simulink model "Emergency_system"  (R2020a)
settings: Solver=ode23tb  StartTime=0.0  StopTime=20  RelTol=1e-4
undefined symbols (not defined in the file or in its folder): ee_sli_rtmsupport, gcbh
libraries: powerlib x10, sps_avr x7, simulink x3, powerlib_meascontrol x2, dspswit3 x1
settings Model: FPTRunName=Active  ExtModeTrigMode=oneshot  ExtModeArmWhenConnect=off  ExtModeAutoUpdateStatusClock=off  Creator=MathWorks  LastModifiedBy=assem
settings SolverCC: ZeroCrossAlgorithm=Adaptive
settings DataIOCC: SaveFormat=Array  SignalLoggingSaveFormat=ModelDataLogs  ReturnWorkspaceOutputs=off  SignalLoggingName=sigsOut  OutputTimes=[0:1/20:10]
settings OptimizationCC: BlockReduction=off  BooleanDataType=off  ExpressionDepthLimit=2147483647  InitFltsAndDblsToZero=on  EfficientMapNaN2IntZero=off  LifeSpan=inf
settings DebuggingCC: UnderspecifiedInitializationDetection=Classic  MergeDetectMultiDrivingBlocksExec=none  CheckExecutionContextPreStartOutputMsg=on  CheckExecutionContextRuntimeOutputMsg=on  SignalResolutionControl=TryResolveAllWithWarning  IgnoredZcDiagnostic=none  MultiTaskDSMMsg=warning  MultiTaskCondExecSysMsg=none  SigSpecEnsureSampleTimeMsg=none  FcnCallInpInsideContextMsg=warning  UnconnectedInputMsg=none  UnconnectedOutputMsg=none  UnconnectedLineMsg=none  StateNameClashWarn=warning  SFUnexpectedBacktrackingDiag=warning  SFNoUnconditionalDefaultTransitionDiag=warning  SFExecutionAtInitializationDiag=none  ArithmeticOperatorsInVariantConditions=warning
settings HardwareCC: ProdBitPerPointer=32  ProdBitPerSizeT=32  ProdBitPerPtrDiffT=32  ProdLargestAtomicFloat=None  ProdIntDivRoundTo=Undefined  ProdEndianess=Unspecified  ProdWordSize=32  ProdHWDeviceType=Specified  TargetUnknown=on
settings ModelReferenceCC: PropagateSignalLabelsOutOfModel=off
settings SFSimCC: SimUseLocalCustomCode=off  CustomCodeUndefinedFunction=UseInterfaceOnly
settings RTWCC: RTWUseLocalCustomCode=off
settings CodeAppCC: StateflowObjectComments=on
settings GRTTargetCC: TargetFcnLib=ansi_tfl_tmw.mat  TargetLangStandard=C89/C90 (ANSI)  CombineOutputUpdateFcns=off  GRTInterface=on
settings ConfigComp: CovMetricSettings=dw  CovHtmlReporting=on  CovSaveCumulativeToWorkspaceVar=on  CovSaveSingleToWorkspaceVar=on  CovExternalEMLEnable=off  CovSFcnEnable=off
settings SimscapeCC: SimscapeNormalizeSystem=off

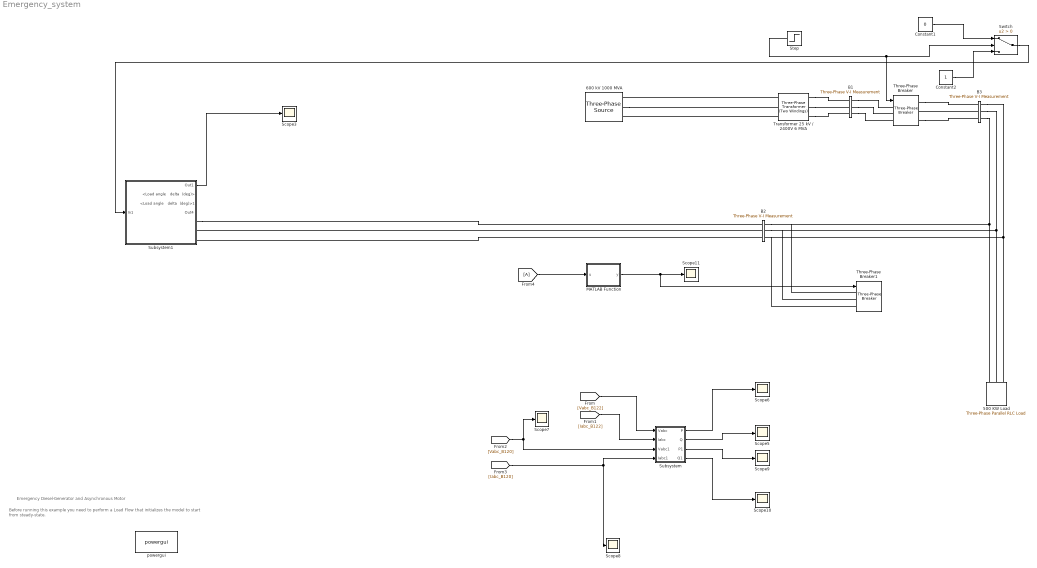
== system Emergency_system ==
  note: Emergency Diesel-Generator and Asynchronous Motor
  note: Before running this example you need to perform a Load Flow that
      | initializes the model to start from steady-state.
  500 KW Load : powerlib/Elements/Three-Phase Parallel RLC Load  LConnTagsString=A|B|C  Configuration=Y (grounded)  NominalVoltage=2400  Vabc=[1e3 1e3 1e3]  Vabcp=[1e3 1e3 1e3]  NominalFrequency=60  UnbalancedPower=off  ActivePower=.5e+006  InductivePower=0  CapacitivePower=0  Pabc=[10e3 9e3 11e3]  QLabc=[100 90 110]  QCabc=[100 90 110]  Pabcp=[10e3 9e3 11e3]  QLabcp=[100 90 110]  QCabcp=[100 90 110]  Measurements=None  LoadType=constant Z
      settings: SourceProductBaseCode=MT,PS
  600 kV 1000 MVA : powerlib/Electrical Sources/Three-Phase Source  InternalConnection=Yg  VoltagePhases=off  Voltage=(13800)*1  PhaseAngle=0.071468  Voltage_phases=[25e3 25e3 25e3]/sqrt(3)  PhaseAngles_phases=[0 -120 +120]  Frequency=60  NonIdealSource=on  SpecifyImpedance=on  Resistance=25^2/1000/10  Inductance=25^2/1000/377  ShortCircuitLevel=1000e6  BaseVoltage=13.8e3  XRratio=7  BusType=swing  Pref=0  Qref=0  Prefabc=[10e3, 10e3, 10e3]  Qrefabc=[0, 0, 0]  Qmin=-Inf  Qmax=Inf
      settings: SourceProductBaseCode=MT,PS
  B1 : powerlib/Measurements/Three-Phase V-I Measurement  VoltageMeasurement=phase-to-ground  SetLabelV=on  LabelV=Vabc_B121  Vpu=off  VpuLL=off  CurrentMeasurement=yes  SetLabelI=on  LabelI=Iabc_B121  Ipu=off  Pbase=100e6  Vbase=120e3  OutputType=Complex  PhasorSimulation=on  PSBequivalent=0
      settings: SourceProductBaseCode=MT,PS
  B2 : powerlib/Measurements/Three-Phase V-I Measurement  VoltageMeasurement=phase-to-ground  SetLabelV=on  LabelV=Vabc_B120  Vpu=off  VpuLL=off  CurrentMeasurement=yes  SetLabelI=on  LabelI=Iabc_B120  Ipu=off  Pbase=100e6  Vbase=120e3  OutputType=Complex  PhasorSimulation=on  PSBequivalent=0
      settings: SourceProductBaseCode=MT,PS
  B3 : powerlib/Measurements/Three-Phase V-I Measurement  VoltageMeasurement=phase-to-ground  SetLabelV=on  LabelV=Vabc_B122  Vpu=off  VpuLL=off  CurrentMeasurement=yes  SetLabelI=on  LabelI=Iabc_B122  Ipu=off  Pbase=100e6  Vbase=120e3  OutputType=Complex  PhasorSimulation=on  PSBequivalent=0
      settings: SourceProductBaseCode=MT,PS
  Constant1 : Constant  Value=0  SampleTime=1
  Constant2 : Constant  SampleTime=1
  MATLAB Function : MATLAB Function  TreatAsAtomicUnit=on
  Scope{3,5..11} (8 alike) : Scope
  Step : Step  Time=4  Before=1  After=0  SampleTime=0
  Subsystem : Subsystem
  Subsystem1 : Subsystem
  Switch : Switch  Criteria=u2 > Threshold
  Three-Phase Breaker : powerlib/Elements/Three-Phase Breaker  InitialState=closed  SwitchA=on  SwitchB=on  SwitchC=on  SwitchTimes="[1/60  5/60]"  External=on  BreakerResistance=0.01  SnubberResistance=1e6  SnubberCapacitance=inf  Measurements=None
  Three-Phase Breaker1 : powerlib/Elements/Three-Phase Breaker  InitialState=closed  SwitchA=on  SwitchB=on  SwitchC=on  SwitchTimes="[1/60  5/60]"  External=on  BreakerResistance=0.01  SnubberResistance=1e6  SnubberCapacitance=inf  Measurements=None
  Transformer 25 kV / 2400V 6 MVA : powerlib/Elements/Three-Phase Transformer (Two Windings)  Winding1Connection=Yg  Winding2Connection=Y  CoreType=Three single-phase transformers  SetSaturation=off  Hysteresis=off  DataFile='hysteresis'  SetInitialFlux=off  Measurements=None  UNITS=pu  NominalPower=[ 6e6 , 60 ]  Winding1=[13.8e3 0.0015 0.03]  Winding2=[2.4e3 0.0015 0.03]  Rm=200  Lm=200  L0=3.7357e-08  Saturation=[0 0;0.005 1.2;1 1.4]  InitialFluxes=[0.022525 -0.022525 0.019709]  BreakLoop=off  DiscreteSolver=Trapezoidal iterative  DataType=off  TransfoNumber=0
      settings: SourceProductBaseCode=MT,PS
  powergui : powerlib/powergui  Priority=2  SimulationMode=Continuous  SampleTime=50e-6  frequency=60  Iterations=50  frequencyindice=60  Pbase=1e6  ErrMax=0.0001  UnitsV=kV  UnitsW=MW  buscounter=0  FunctionMessages=off  echomessages=off  EnableUseOfTLC=off  CurrentSourceSwitches=off  DisableSnubberDevices=on  DisableRonSwitches=off  DisableVfSwitches=off  DisplayEquations=off  AutomaticDiscreteSolvers=off  SolverType=Tustin  Interpol=off  ExternalGateDelay=off  methode=off  Ts=0  x0status=blocks  SPID=on  SwTol=0  HookPort=off  NonlinearTolerance=1e-4  nMaxIteration=100  ContinueOnMaxIteration=off  RestoreLinks=warning  ResistiveCurrentMeasurement=off  Frange=logspace(0,3,50)  Ylog=off  Xlog=off  ShowGrid=off  save=off  variable=ZData  structure=0  ZoomFFT=on  StartTime=0.0  cycles=2  DisplayStyle=off  fundamental=60  FreqAxis=off  MaxFrequency=1000  frequencyindicesteady=1  RmsSteady=1  display=off
  wires:
  Step/1 -> Three-Phase Breaker/1, Switch/2
  Constant2/1 -> Switch/3
  Constant1/1 -> Switch/1
  [Vabc_B120] -> Subsystem/3(Vabc1), Scope7/1
  [Iabc_B120] -> Subsystem/4(Iabc1), Scope8/1
  [A] -> MATLAB Function/1(u)
  MATLAB Function/1(y) -> Three-Phase Breaker1/1, Scope11/1
  [Vabc_B122] -> Subsystem/1(Vabc)
  [Iabc_B122] -> Subsystem/2(Iabc)
  Subsystem/1(P) -> Scope6/1
  Subsystem/2(Q) -> Scope5/1
  Subsystem/3(P1) -> Scope9/1
  Subsystem/4(Q1) -> Scope10/1
  Switch/1 -> Subsystem1/1(In1)
  Subsystem1/1(Out1) -> Scope3/1
  connections:
  Transformer 25 kV / 2400V 6 MVA/LConn1 -- 600 kV 1000 MVA/RConn1
  600 kV 1000 MVA/RConn2 -- Transformer 25 kV / 2400V 6 MVA/LConn2
  Transformer 25 kV / 2400V 6 MVA/LConn3 -- 600 kV 1000 MVA/RConn3
  Transformer 25 kV / 2400V 6 MVA/RConn1 -- B1/LConn1
  Transformer 25 kV / 2400V 6 MVA/RConn2 -- B1/LConn2
  Transformer 25 kV / 2400V 6 MVA/RConn3 -- B1/LConn3
  B1/RConn1 -- Three-Phase Breaker/LConn1
  B1/RConn2 -- Three-Phase Breaker/LConn2
  B1/RConn3 -- Three-Phase Breaker/LConn3
  B3/LConn2 -- Three-Phase Breaker/RConn2
  Three-Phase Breaker/RConn1 -- B3/LConn1
  Three-Phase Breaker/RConn3 -- B3/LConn3
  B3/RConn1 -- Three-Phase Breaker1/LConn3 -- B2/RConn3 -- 500 KW Load/LConn3
  B3/RConn2 -- Three-Phase Breaker1/LConn2 -- B2/RConn2 -- 500 KW Load/LConn2
  B3/RConn3 -- Three-Phase Breaker1/LConn1 -- B2/RConn1 -- 500 KW Load/LConn1
  Subsystem1/RConn1 -- B2/LConn1
  B2/LConn2 -- Subsystem1/RConn2
  B2/LConn3 -- Subsystem1/RConn3

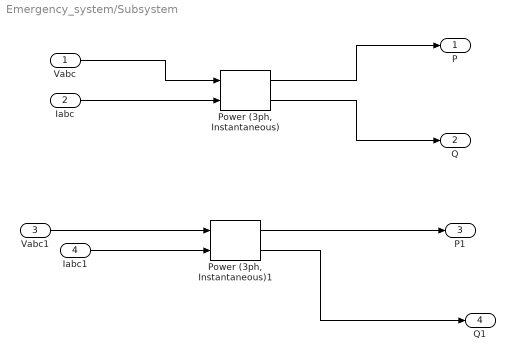
== system Emergency_system/Subsystem ==
  Vabc : Inport
  Iabc : Inport  Port=2
  Vabc1 : Inport  Port=3
  Iabc1 : Inport  Port=4
  "Power (3ph, Instantaneous)" : powerlib_meascontrol/Measurements/Power (3ph, Instantaneous)
  "Power (3ph, Instantaneous)1" : powerlib_meascontrol/Measurements/Power (3ph, Instantaneous)
  P : Outport
  Q : Outport  Port=2
  P1 : Outport  Port=3
  Q1 : Outport  Port=4
  wires:
  "Power (3ph, Instantaneous)1"/1 -> P1/1
  Vabc/1 -> "Power (3ph, Instantaneous)"/1
  "Power (3ph, Instantaneous)"/1 -> P/1
  Iabc1/1 -> "Power (3ph, Instantaneous)1"/2
  "Power (3ph, Instantaneous)1"/2 -> Q1/1
  Iabc/1 -> "Power (3ph, Instantaneous)"/2
  "Power (3ph, Instantaneous)"/2 -> Q/1
  Vabc1/1 -> "Power (3ph, Instantaneous)1"/1

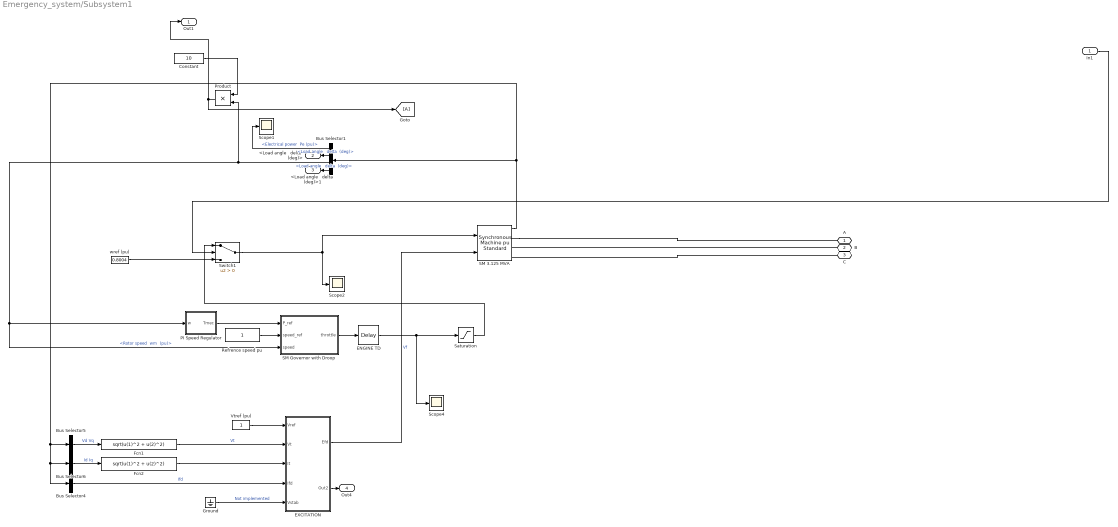
== system Emergency_system/Subsystem1 ==
  In1 : Inport
  Bus Selector1 : BusSelector  OutputSignals="Mechanical.Electrical power  Pe (pu),Load angle   delta  (deg),Mechanical.Rotor speed  wm  (pu),Load angle   delta  (deg)"
  Bus Selector4 : BusSelector  OutputSignals="dq0 components.Field current  ifd (pu)"  OutputAsBus=on
  Bus Selector5 : BusSelector  OutputSignals="dq0 components.Stator voltage  vd (pu),dq0 components.Stator voltage  vq (pu)"  OutputAsBus=on
  Bus Selector6 : BusSelector  OutputSignals="dq0 components.Stator current  id (pu),dq0 components.Stator current  iq (pu)"  OutputAsBus=on
  Constant : Constant  Value=10
  ENGINE TD : TransportDelay  BufferSize=19456
  EXCITATION : Subsystem  Variant=on  VariantControlMode=Label  LabelModeActiveChoice=Variant1
      settings: AttributesFormatString=%<BlockChoice>
  Fcn1 : Fcn  Expr=sqrt(u(1)^2 + u(2)^2)
  Fcn2 : Fcn  Expr=sqrt(u(1)^2 + u(2)^2)
  Ground : Ground
  PI Speed Regulator : Subsystem
  Product : Product
  Refrence speed pu : Constant
  SM 3.125 MVA : powerlib/Machines/Synchronous Machine pu Standard  PresetModel=No  MechanicalLoad=Mechanical power Pm  ShowDetailedParameters=on  RotorType=Salient-pole  Units=per unit standard parameters  MeasurementBus=off  NominalParameters=[700e3 2400 60]  Reactances1=[ 31 32 33 34 35 36 37 ]  Reactances2=[1.56 0.296 0.177 1.06 0.277 0.052]  dAxisTimeConstants=Short-circuit  qAxisTimeConstants=Open-circuit  TimeConstants1=[]  TimeConstants2=[]  TimeConstants3=[]  TimeConstants4=[]  TimeConstants5=[ 3.7, 0.05, 0.05 ]  TimeConstants6=[ 8.0, 0.03, 0.3371, 0.0295 ]  TimeConstants7=[0.08 0.012 0.012]  TimeConstants8=[]  StatorResistance=0.0036  Mechanical=[1.07 0 2]  PolePairs=2  InitialConditions=[0 0 0 0 0 0 0 0 1]  SetSaturation=off  Saturation=[0.211 0.418 1.0 1.25 1.72 3.35 ;0.25 0.50 1.0 1.1 1.2 1.4]  LoadFlowParameters=[1 0 0 0]  TsPowergui=0  TsBlock=-1  IterativeModel=Trapezoidal non iterative  IterativeDiscreteModel=Trapezoidal non iterative  BusType=swing  Pref=0  Qref=0  Qmin=-Inf  Qmax=Inf  PLF=0  QLF=0
      settings: AttributesFormatString=\n\n  SourceProductBaseCode=MT,PS
  SM Governor with Droop : Subsystem  AncestorBlock=eeSmGovernor/SM Governor with Droop  LoadFcn=ee_sli_rtmsupport( 'loadfcn', gcbh );  mask(SM Governor with Droop){droop_percentage=5, T_G=0.0001, pu_throttle0=0.8}
      mask prompts: droop_percentage "physmod:ee:library:comments:control:eeSmGovernor:PercentageDroop_MP"; T_G "physmod:ee:library:comments:control:eeSmGovernor:TimeConstantOfGovernors_MP"; pu_throttle0 "physmod:ee:library:comments:control:eeSmGovernor:InitialThrottlePositionpu_MP"
      mask help: physmod:ee:library:comments:control:eeSmGovernor:SMGovernorWithDroop_MD
      settings: CopyFcn=ee_sli_rtmsupport( 'copyfcn', gcbh );  DeleteFcn=ee_sli_rtmsupport( 'deletefcn', gcbh );  ModelCloseFcn=ee_sli_rtmsupport( 'modelclosefcn', gcbh );  PostSaveFcn=ee_sli_rtmsupport( 'postsavefcn', gcbh );  PreCopyFcn=ee_sli_rtmsupport( 'precopyfcn', gcbh );  OpenFcn=ee_sli_rtmsupport( 'openfcn', gcbh );  CloseFcn=ee_sli_rtmsupport( 'closefcn', gcbh );  PreDeleteFcn=ee_sli_rtmsupport( 'predeletefcn', gcbh );
      mask Help: web(nesl_help(gcbh))
  Saturation : Saturate
  Scope1 : Scope
  Scope2 : Scope
  Scope4 : Scope
  Switch1 : Switch  Criteria=u2 > Threshold
  "Vtref (pu) " : Constant
  wref (pu) : Constant  Value=0.8004
  A : PMIOPort  Side=Right
  B : PMIOPort  Port=2  Side=Right
  C : PMIOPort  Port=3  Side=Right
  Out1 : Outport
  <Load angle   delta  (deg)> : Outport  Port=2
  <Load angle   delta  (deg)>1 : Outport  Port=3
  Out4 : Outport  Port=4
  wires:
  ENGINE TD/1 -> Scope4/1, Saturation/1
  SM 3.125 MVA/1 -> Bus Selector5/1, Bus Selector6/1, Bus Selector4/1, Bus Selector1/1
  Ground/1 -> EXCITATION/5(Vstab)  "Not implemented"
  PI Speed Regulator/1(Tmec) -> SM Governor with Droop/1(P_ref)
  Bus Selector1/3 -> PI Speed Regulator/1(w), SM Governor with Droop/3(speed), Product/2  "<Rotor speed  wm  (pu)>"
  In1/1 -> Switch1/2
  Bus Selector1/1 -> Scope1/1  "<Electrical power  Pe (pu)>"
  Saturation/1 -> Switch1/1
  Bus Selector1/2 -> <Load angle   delta  (deg)>/1  "<Load angle   delta  (deg)>"
  wref (pu)/1 -> Switch1/3
  Product/1 -> Out1/1, [A]
  Bus Selector6/1 -> Fcn2/1  "Id Iq"
  Refrence speed pu/1 -> SM Governor with Droop/2(speed_ref)
  SM Governor with Droop/1(throttle) -> ENGINE TD/1
  EXCITATION/2(Out2) -> Out4/1
  Bus Selector1/4 -> <Load angle   delta  (deg)>1/1  "<Load angle   delta  (deg)>"
  Bus Selector4/1 -> EXCITATION/4(Ifd)  "Ifd"
  Bus Selector5/1 -> Fcn1/1  "Vd Vq"
  Switch1/1 -> Scope2/1, SM 3.125 MVA/1
  "Vtref (pu) "/1 -> EXCITATION/1(Vref)
  Constant/1 -> Product/1
  Fcn2/1 -> EXCITATION/3(It)
  Fcn1/1 -> EXCITATION/2(Vt)  "Vt"
  EXCITATION/1(Efd) -> SM 3.125 MVA/2  "Vf"
  connections:
  B/RConn1 -- SM 3.125 MVA/RConn2
  SM 3.125 MVA/RConn1 -- A/RConn1
  C/RConn1 -- SM 3.125 MVA/RConn3

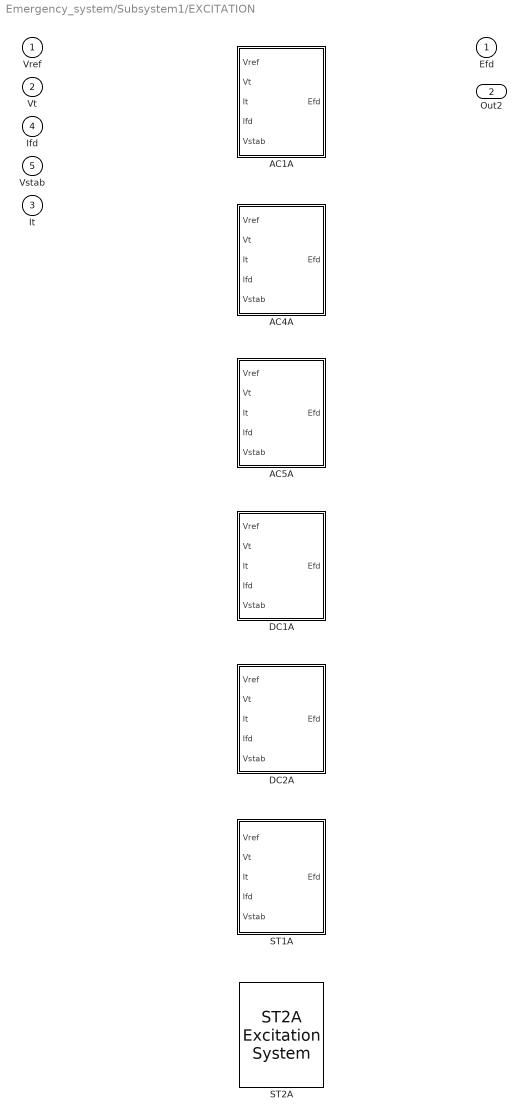
== system Emergency_system/Subsystem1/EXCITATION ==
  Vref : Inport
  Vt : Inport  Port=2
  It : Inport  Port=3
  Ifd : Inport  Port=4
  Vstab : Inport  Port=5
  AC1A : Subsystem  VariantControl=Variant1
  AC4A : Subsystem  VariantControl=Variant2
  AC5A : Subsystem  VariantControl=Variant3
  DC1A : Subsystem  VariantControl=Variant4
  DC2A : Subsystem  VariantControl=Variant5
  ST1A : Subsystem  VariantControl=Variant6
  ST2A : sps_avr/ST2A Excitation System  VariantControl=Variant7  Tr=20e-3  KaTa=[120 0.15]  VRminmax=[0 1.0]  KfTf=[0.05 1.0]  KeTe=[1.0 0.5]  KI=8.0  Kp=4.88  Xd=1.56  Kc=1.82  v0=[1,1.42734]  I0=0.2739  TsBlock=-2
      settings: SourceProductBaseCode=MT,PS
  Efd : Outport  VectorParamsAs1DForOutWhenUnconnected=off
  Out2 : Outport  Port=2

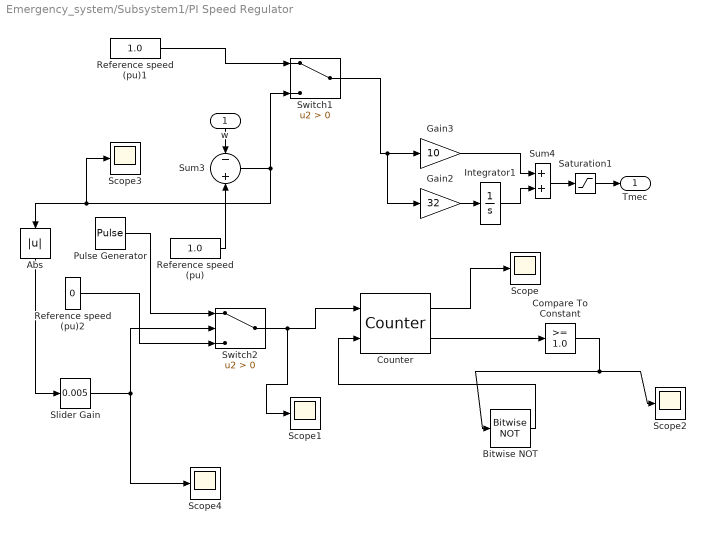
== system Emergency_system/Subsystem1/PI Speed Regulator ==
  w : Inport
  Abs : Abs
  Bitwise NOT : simulink/Logic and Bit Operations/Bitwise Operator  logicop=NOT  UseBitMask=off  BitMask=bin2dec('11011001')  BitMaskRealWorld=Stored Integer
  Compare To Constant : simulink/Logic and Bit Operations/Compare To Constant  relop=>=  const=1.0  OutDataTypeStr=boolean
  Counter : dspswit3/Counter  Direction=Up  CountEvent=Rising edge  CounterSize=User defined  MaxCount=255  InitialCount=0  Output=Count and Hit  HitValue=32  ResetInput=on  SamplesPerFrame=1  Ts=1  CntDtype=double  HitDtype=Logical
  Gain2 : Gain  Gain=32  SaturateOnIntegerOverflow=on  OutDataTypeStr=Inherit: Same as input  ParamDataTypeStr=Inherit: Same as input
  Gain3 : Gain  Gain=10  SaturateOnIntegerOverflow=on  OutDataTypeStr=Inherit: Same as input  ParamDataTypeStr=Inherit: Same as input
  Integrator1 : Integrator  InitialCondition=0.8024  LimitOutput=on  UpperSaturationLimit=1  LowerSaturationLimit=0  ZeroCross=off
  Pulse Generator : DiscretePulseGenerator  PulseType=Time based  Period=5  PulseWidth=2
  Reference speed (pu) : Constant  Value=1.0
  Reference speed (pu)1 : Constant  Value=1.0
  Reference speed (pu)2 : Constant  Value=0
  Saturation1 : Saturate  UpperLimit=1  LowerLimit=0  ZeroCross=off
  Scope{,1..4} (5 alike) : Scope
  Slider Gain : simulink/Math Operations/Slider Gain  gain=0.005  low=0  high=2
  Sum3 : Sum  Inputs=-+  InputSameDT=on  SaturateOnIntegerOverflow=on  OutDataTypeStr=Inherit: Same as first input
  Sum4 : Sum  InputSameDT=on  SaturateOnIntegerOverflow=on  OutDataTypeStr=Inherit: Same as first input
  Switch1 : Switch  Criteria=u2 > Threshold
  Switch2 : Switch  Criteria=u2 > Threshold
  Tmec : Outport  VectorParamsAs1DForOutWhenUnconnected=off
  wires:
  Gain3/1 -> Sum4/1
  Gain2/1 -> Integrator1/1
  Integrator1/1 -> Sum4/2
  Reference speed (pu)/1 -> Sum3/2
  Sum4/1 -> Saturation1/1
  w/1 -> Sum3/1
  Saturation1/1 -> Tmec/1
  Reference speed (pu)1/1 -> Switch1/1
  Pulse Generator/1 -> Switch2/1
  Switch2/1 -> Scope1/1, Counter/1
  Bitwise NOT/1 -> Counter/2
  Reference speed (pu)2/1 -> Switch2/3
  Sum3/1 -> Scope3/1, Abs/1, Switch1/3
  Switch1/1 -> Gain3/1, Gain2/1
  Counter/2 -> Compare To Constant/1
  Compare To Constant/1 -> Bitwise NOT/1, Scope2/1
  Counter/1 -> Scope/1
  Slider Gain/1 -> Switch2/2, Scope4/1
  Abs/1 -> Slider Gain/1

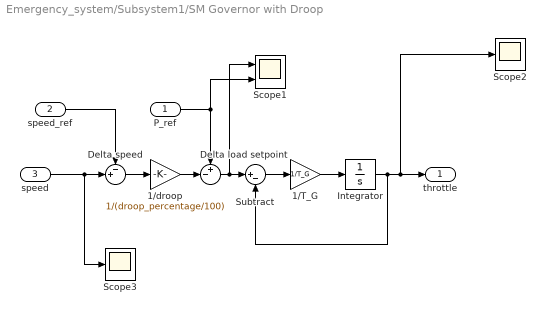
== system Emergency_system/Subsystem1/SM Governor with Droop ==
  P_ref : Inport
  speed_ref : Inport  Port=2
  speed : Inport  Port=3
  1/T_G : Gain  Gain=1/T_G
  1/droop : Gain  Gain=1/(droop_percentage/100)
  Delta load setpoint : Sum  Inputs=+-|
  Delta speed : Sum  Inputs=-+|
  Integrator : Integrator  InitialCondition=pu_throttle0
  Scope1 : Scope  NumInputPorts=2
  Scope2 : Scope
  Scope3 : Scope
  Subtract : Sum  Inputs=|+-
  throttle : Outport  VectorParamsAs1DForOutWhenUnconnected=off
  wires:
  Integrator/1 -> Scope2/1, throttle/1, Subtract/2
  1/T_G/1 -> Integrator/1
  Delta speed/1 -> 1/droop/1
  Delta load setpoint/1 -> Scope1/1, Subtract/1
  speed_ref/1 -> Delta speed/1
  P_ref/1 -> Scope1/2, Delta load setpoint/1
  Subtract/1 -> 1/T_G/1
  speed/1 -> Delta speed/2, Scope3/1
  1/droop/1 -> Delta load setpoint/2

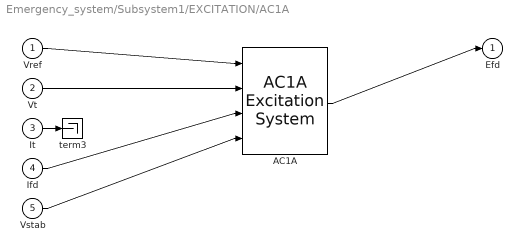
== system Emergency_system/Subsystem1/EXCITATION/AC1A ==
  Vref : Inport
  Vt : Inport  Port=2
  It : Inport  Port=3
  Ifd : Inport  Port=4
  Vstab : Inport  Port=5
  AC1A : sps_avr/AC1A Excitation System  Tr=20e-3  KaTa=[400 0.02]  VAminmax=[-14.5 14.5]  VRminmax=[-5.43 6.03]  KfTf=[0.03 1.0]  TbTc=[0 0]  KeTe=[1.0 0.80]  Ve12=[4.18 3.14]  SeVe12=[0.10 0.03]  Kd=0.38  Kc=0.20  v0=[1 1.4273]  TsBlock=-2
      settings: SourceProductBaseCode=MT,PS
  term3 : Terminator
  Efd : Outport  VectorParamsAs1DForOutWhenUnconnected=off
  wires:
  It/1 -> term3/1
  AC1A/1 -> Efd/1
  Vstab/1 -> AC1A/4
  Ifd/1 -> AC1A/3
  Vt/1 -> AC1A/2
  Vref/1 -> AC1A/1

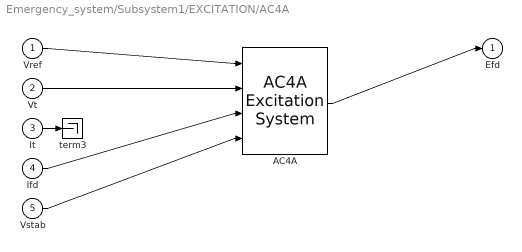
== system Emergency_system/Subsystem1/EXCITATION/AC4A ==
  Vref : Inport
  Vt : Inport  Port=2
  It : Inport  Port=3
  Ifd : Inport  Port=4
  Vstab : Inport  Port=5
  AC4A : sps_avr/AC4A Excitation System  Tr=20e-3  KaTa=[200 0.015]  VIminmax=[-10 10]  VRminmax=[-4.53 5.64]  TbTc=[10 1.0]  Kc=0  v0=[1,1.42734]  TsBlock=-2
      settings: SourceProductBaseCode=MT,PS
  term3 : Terminator
  Efd : Outport  VectorParamsAs1DForOutWhenUnconnected=off
  wires:
  It/1 -> term3/1
  AC4A/1 -> Efd/1
  Vstab/1 -> AC4A/4
  Ifd/1 -> AC4A/3
  Vt/1 -> AC4A/2
  Vref/1 -> AC4A/1

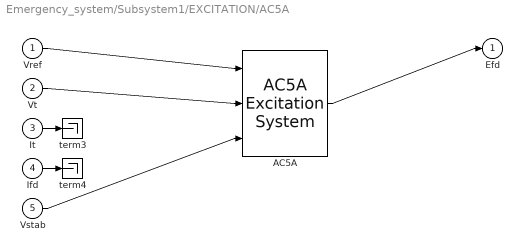
== system Emergency_system/Subsystem1/EXCITATION/AC5A ==
  Vref : Inport
  Vt : Inport  Port=2
  It : Inport  Port=3
  Ifd : Inport  Port=4
  Vstab : Inport  Port=5
  AC5A : sps_avr/AC5A Excitation System  Tr=20e-3  KaTa=[100 0.02]  VRminmax=[-7.3 7.3]  KfTf=[0.03 1 0 0]  KeTe=[1.0 0.02]  Efd12=[5.6 0.75*5.6]  SeEfd12=[0.86 0.5]  v0=[1,1.42734]  TsBlock=-2
      settings: SourceProductBaseCode=MT,PS
  term3 : Terminator
  term4 : Terminator
  Efd : Outport  VectorParamsAs1DForOutWhenUnconnected=off
  wires:
  Ifd/1 -> term4/1
  It/1 -> term3/1
  AC5A/1 -> Efd/1
  Vstab/1 -> AC5A/3
  Vt/1 -> AC5A/2
  Vref/1 -> AC5A/1

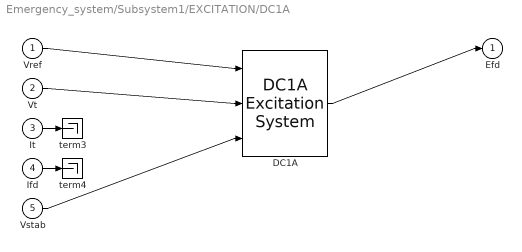
== system Emergency_system/Subsystem1/EXCITATION/DC1A ==
  Vref : Inport
  Vt : Inport  Port=2
  It : Inport  Port=3
  Ifd : Inport  Port=4
  Vstab : Inport  Port=5
  DC1A : sps_avr/DC1A Excitation System  Tr=20e-3  KaTa=[46 0.06]  VRminmax=[-0.9 1.0]  KfTf=[0.05 1.5]  TbTc=[0 0]  KeTe=[0.05 0.46]  Efd12=[3.1 2.3]  SeEfd12=[0.33 0.10]  v0=[1,1.42734]  TsBlock=-2
      settings: SourceProductBaseCode=MT,PS
  term3 : Terminator
  term4 : Terminator
  Efd : Outport  VectorParamsAs1DForOutWhenUnconnected=off
  wires:
  Ifd/1 -> term4/1
  It/1 -> term3/1
  DC1A/1 -> Efd/1
  Vstab/1 -> DC1A/3
  Vt/1 -> DC1A/2
  Vref/1 -> DC1A/1

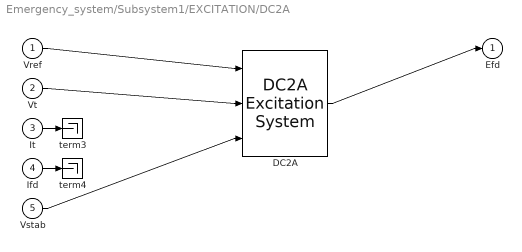
== system Emergency_system/Subsystem1/EXCITATION/DC2A ==
  Vref : Inport
  Vt : Inport  Port=2
  It : Inport  Port=3
  Ifd : Inport  Port=4
  Vstab : Inport  Port=5
  DC2A : sps_avr/DC2A Excitation System  Tr=20e-3  KaTa=[46 0.06]  VRminmax=[-4.9 4.95]  KfTf=[0.05 1.5]  TbTc=[0 0]  KeTe=[0.05 0.46]  Efd12=[3.05 2.29]  SeEfd12=[0.279 0.117]  v0=[1,1.42734]  TsBlock=-2
      settings: SourceProductBaseCode=MT,PS
  term3 : Terminator
  term4 : Terminator
  Efd : Outport  VectorParamsAs1DForOutWhenUnconnected=off
  wires:
  Ifd/1 -> term4/1
  It/1 -> term3/1
  DC2A/1 -> Efd/1
  Vstab/1 -> DC2A/3
  Vt/1 -> DC2A/2
  Vref/1 -> DC2A/1

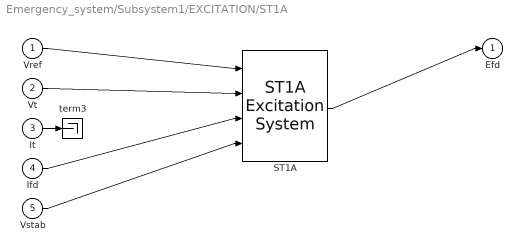
== system Emergency_system/Subsystem1/EXCITATION/ST1A ==
  Vref : Inport
  Vt : Inport  Port=2
  It : Inport  Port=3
  Ifd : Inport  Port=4
  Vstab : Inport  Port=5
  ST1A : sps_avr/ST1A Excitation System  Tr=20e-3  KaTa=[210 0.001]  VIminmax=[-999 999]  VAminmax=[-999 999]  VRminmax=[-6.0 6.43]  KfTf=[0.001 1]  TbTc=[0 0 0 0]  KLR=1  ILR=2  Kc=0.038  v0=[1,1.42734]  TsBlock=-2
      settings: SourceProductBaseCode=MT,PS
  term3 : Terminator
  Efd : Outport  VectorParamsAs1DForOutWhenUnconnected=off
  wires:
  It/1 -> term3/1
  ST1A/1 -> Efd/1
  Vstab/1 -> ST1A/4
  Ifd/1 -> ST1A/3
  Vt/1 -> ST1A/2
  Vref/1 -> ST1A/1

== matlab function Emergency_system/MATLAB Function ==
  data: u input; y output
function y = fcn(u)
if (u>60.5)
    y=1;
elseif (u<57.5)
   
    y=0;
    
else
    y=1;
end
end
